simulink subsystem "TPhase_Vector_Generator"  (R2024b)
settings: Solver=VariableStepAuto  StartTime=0.0  StopTime=10.0  RelTol=1e-3
settings Model: Creator=antoinedaniel  LastModifiedBy=antoinedaniel

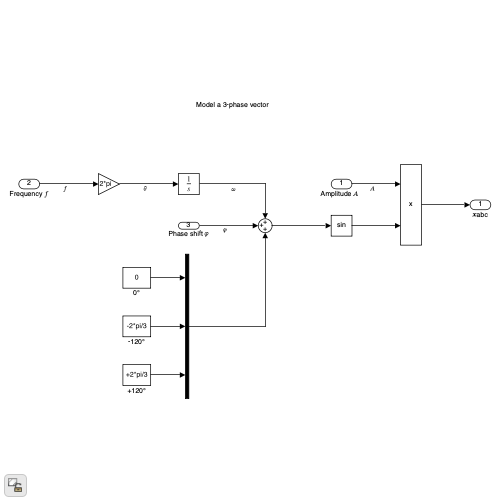
[thumbnail: Simulink's stored preview of the top-level diagram]
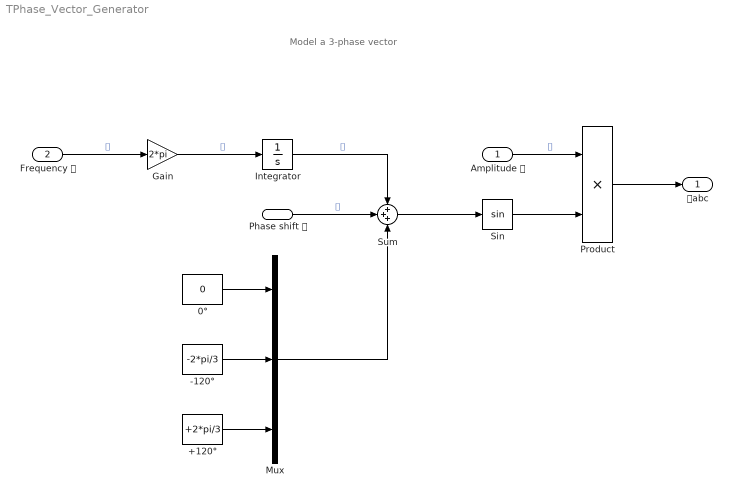
== system TPhase_Vector_Generator ==
  note: Model a 3-phase vector
  "Amplitude 𝐴  " : Inport
  Frequency 𝑓 : Inport  Port=2
  Phase shift 𝜑 : Inport  Port=3
  +120° : Constant  Value=+2*pi/3
  -120° : Constant  Value=-2*pi/3
  0° : Constant  Value=0
  Gain : Gain  Gain=2*pi
  Integrator : Integrator
  Mux : Mux  Inputs=3
  Product : Product
  Sin : Trigonometry
  Sum : Sum  Inputs=+++
  𝒙abc : Outport
  wires:
  -120°/1 -> Mux/2
  0°/1 -> Mux/1
  +120°/1 -> Mux/3
  Frequency 𝑓/1 -> Gain/1  "𝑓"
  Gain/1 -> Integrator/1  "𝜃"
  Phase shift 𝜑/1 -> Sum/2  "𝜑"
  Mux/1 -> Sum/3
  Integrator/1 -> Sum/1  "𝜔"
  Sum/1 -> Sin/1
  "Amplitude 𝐴  "/1 -> Product/1  "𝐴"
  Sin/1 -> Product/2
  Product/1 -> 𝒙abc/1
